simulink model "Assignment_2"  (R2022b)
settings: Solver=FixedStepAuto  StartTime=0.0  StopTime=10.0  FixedStep=1e-3  RelTol=1e-3  EnableMultiTasking=on
undefined symbols (not defined in the file): D0, D1, D10, D11, D12, D13, D2, D3, D5, D6, D8, D9, PTA0, PTA1, PTA2, PTB9, PTC16, PTC17, PTC2, PTC4, PTD0, PTD1, PTD2, PTD3
libraries: frdmk64flib x12
settings Model: ExtModeTrigDuration=5  Creator=aldenluscher  LastModifiedBy=andre
settings OptimizationCC: EnhancedBackFolding=on  PassReuseOutputArgsAs=Individual arguments  ZeroExternalMemoryAtStartup=off  ZeroInternalMemoryAtStartup=off  MaxStackSize=64  OptimizeBlockOrder=speed  DifferentSizesBufferReuse=on  OptimizationCustomize=off  EfficientTunableParamExpr=on
settings DebuggingCC: ParameterTunabilityLossMsg=error
settings HardwareCC: ProdBitPerPointer=32  ProdBitPerSizeT=32  ProdBitPerPtrDiffT=32  ProdLargestAtomicInteger=Long  ProdLargestAtomicFloat=Double  ProdWordSize=32  ProdHWDeviceType=ARM Compatible->ARM Cortex
settings SFSimCC: MATLABDynamicMemAlloc=off
settings RTWCC: Description=Embedded Coder  SystemTargetFile=ert.tlc  HardwareBoard=NXP FRDM-K64F  TLCOptions="-aInlineSetEventsForThisBaseRateFcn=TLC_FALSE -aSuppressMultiTaskScheduler=TLC_FALSE  -aRateBasedStepFcn=0"  TemplateMakefile=ert_default_tmf  Toolchain=GNU Tools for ARM Embedded Processors
settings CodeAppCC: ForceParamTrailComments=on  IgnoreCustomStorageClasses=off  OperatorAnnotations=on  SimulinkDataObjDesc=on  SFDataObjDesc=on  InsertBlockDesc=on
settings ERTTargetCC: ExtModeTransport=4  ExtModeMexFile=sendToCommService

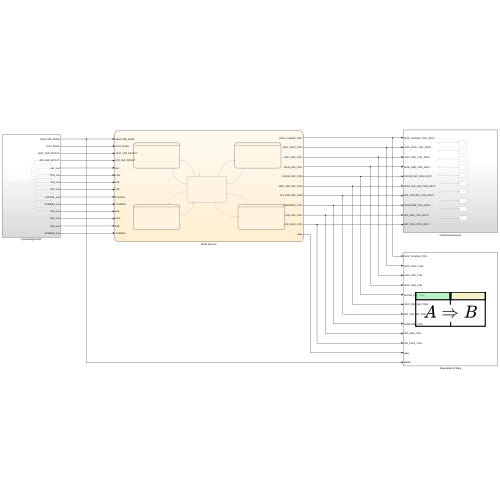
[thumbnail: Simulink's stored preview of the top-level diagram]
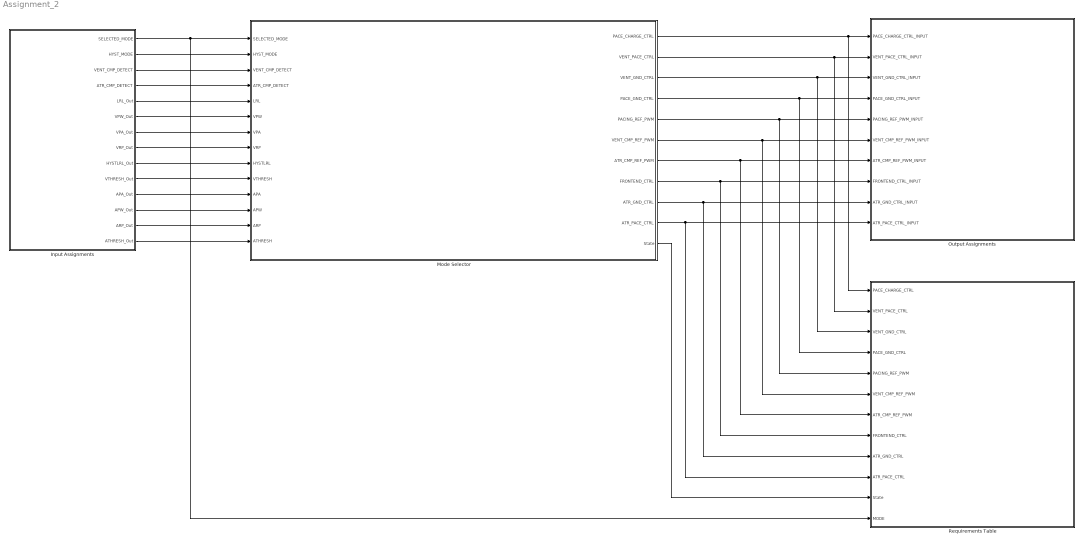
== system Assignment_2 ==
  Input Assignments : Subsystem
  Mode Selector : Stateflow chart  TreatAsAtomicUnit=on
      settings: PortSchema="{\"entries\":[{\"content\":{\"sides\":[{\"content\":{\"connectorIds\":[\"In7\",\"In9\",\"In6\",\"In14\",\"In8\",\"In3\",\"In4\",\"In2\",\"In5\",\"In1\",\"In10\",\"In11\",\"In12\",\"In13\"]},\"type\":\"ConnectorPlacement.EquallySpacedRectSide\",\"uuid\":\"804be3be-5f9e-4b62-b5c8-dc084235daae\"},{\"content\":{\"connectorIds\":[\"Out1\",\"Out2\",\"Out3\",\"Out4\",\"Out5\",\"Out6\",\"Out11\",\"Out7\",\"Out8\",\"Out9\",\"Out10\"],\"side\":\"RIGHT\"},\"type\":\"ConnectorPlacement.EquallySpacedRectSide\",\"uuid\":\"906acfdb-1dc8-44fd-8d51-f28f98719a27\"},{\"content\":{\"connectorIds\":[],\"side\":\"TOP\"},\"type\":\"ConnectorPlacement.EquallySpacedRectSide\",\"uuid\":\"8d057b55-2cbd-487f-8484-177f9fa59c90\"}]},\"type\":\"ConnectorPlacement.EquallySpacedConnector\",\"uuid\":\"d5bd6f86-9a36-412f-a1f0-e96663509123\"}],\"packageUris\":[\"http://schema.mathworks.com/mf0/Connector/R2020b\"],\"version\":\"1.0\"}"
  Output Assignments : Subsystem
  Requirements Table : Requirements Table  TreatAsAtomicUnit=on
  wires:
  Mode Selector/4(PACE_GND_CTRL) -> Requirements Table/4(PACE_GND_CTRL), Output Assignments/4(PACE_GND_CTRL_INPUT)
  Mode Selector/7(FRONTEND_CTRL) -> Output Assignments/8(FRONTEND_CTRL_INPUT), Requirements Table/8(FRONTEND_CTRL)
  Mode Selector/5(PACING_REF_PWM) -> Requirements Table/5(PACING_REF_PWM), Output Assignments/5(PACING_REF_PWM_INPUT)
  Mode Selector/1(PACE_CHARGE_CTRL) -> Requirements Table/1(PACE_CHARGE_CTRL), Output Assignments/1(PACE_CHARGE_CTRL_INPUT)
  Mode Selector/3(VENT_GND_CTRL) -> Requirements Table/3(VENT_GND_CTRL), Output Assignments/3(VENT_GND_CTRL_INPUT)
  Mode Selector/6(VENT_CMP_REF_PWM) -> Requirements Table/6(VENT_CMP_REF_PWM), Output Assignments/6(VENT_CMP_REF_PWM_INPUT)
  Mode Selector/2(VENT_PACE_CTRL) -> Requirements Table/2(VENT_PACE_CTRL), Output Assignments/2(VENT_PACE_CTRL_INPUT)
  Mode Selector/8(ATR_GND_CTRL) -> Output Assignments/9(ATR_GND_CTRL_INPUT), Requirements Table/9(ATR_GND_CTRL)
  Mode Selector/9(ATR_PACE_CTRL) -> Output Assignments/10(ATR_PACE_CTRL_INPUT), Requirements Table/10(ATR_PACE_CTRL)
  Mode Selector/10(State) -> Requirements Table/11(State)
  Mode Selector/11(ATR_CMP_REF_PWM) -> Requirements Table/7(ATR_CMP_REF_PWM), Output Assignments/7(ATR_CMP_REF_PWM_INPUT)
  Input Assignments/1(SELECTED_MODE) -> Requirements Table/12(MODE), Mode Selector/7(SELECTED_MODE)
  Input Assignments/2(HYST_MODE) -> Mode Selector/9(HYST_MODE)
  Input Assignments/3(VENT_CMP_DETECT) -> Mode Selector/6(VENT_CMP_DETECT)
  Input Assignments/4(ATR_CMP_DETECT) -> Mode Selector/14(ATR_CMP_DETECT)
  Input Assignments/5(LRL_Out) -> Mode Selector/8(LRL)
  Input Assignments/6(VPW_Out) -> Mode Selector/3(VPW)
  Input Assignments/7(VPA_Out) -> Mode Selector/4(VPA)
  Input Assignments/8(VRP_Out) -> Mode Selector/2(VRP)
  Input Assignments/9(HYSTLRL_Out) -> Mode Selector/5(HYSTLRL)
  Input Assignments/10(VTHRESH_Out) -> Mode Selector/1(VTHRESH)
  Input Assignments/11(APA_Out) -> Mode Selector/10(APA)
  Input Assignments/12(APW_Out) -> Mode Selector/11(APW)
  Input Assignments/13(ARP_Out) -> Mode Selector/12(ARP)
  Input Assignments/14(ATHRESH_Out) -> Mode Selector/13(ATHRESH)

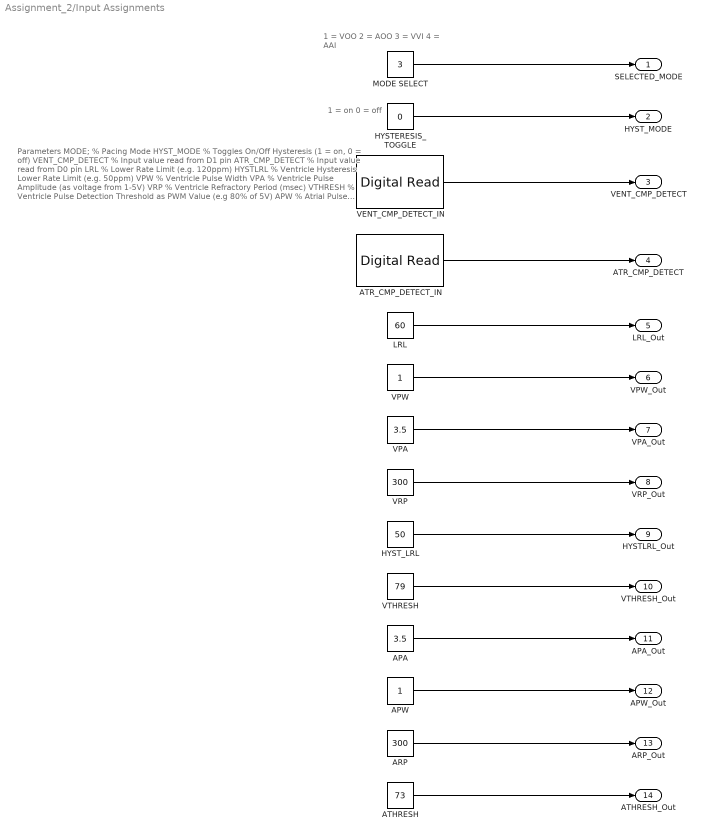
== system Assignment_2/Input Assignments ==
  note: Parameters
      | MODE; 					% Pacing Mode
      | HYST_MODE 			% Toggles On/Off Hysteresis (1 = on, 0 = off)
      | VENT_CMP_DETECT 	% Input value read from D1 pin
      | ATR_CMP_DETECT 		% Input value read from D0 pin
      | LRL 		%  Lower Rate Limit (e.g. 120ppm)
      | HYSTLRL	% Ventricle Hysteresis Lower Rate Limit (e.g. 50ppm)
      | VPW		% Ventricle Pulse Width
      | VPA 		% Ventricle Pulse Amplitude (as voltage from 1-5V)
      | VRP		% Ventricle Refractory Period (msec)
      | VTHRESH 	% Ventricle Pulse Detection Threshold as PWM Value (e.g 80% of 5V)
      | APW		% Atrial Pulse Width
      | APA 		% Atrial Pulse Amplitude (as voltage from 1-5V)
      | ARP 		% Atrial Refractory Period (msec)
      | ATHRESH 	% Atrial Pulse Detection Threshold as a PWM Value (e.g. 80% of 5V)
  note: 1 = VOO
      | 2 = AOO
      | 3 = VVI
      | 4 = AAI
  note: 1 = on
      | 0 = off
  APA : Constant  Value=3.5
  APW : Constant
  ARP : Constant  Value=300
  ATHRESH : Constant  Value=73
  ATR_CMP_DETECT_IN : frdmk64flib/Digital Read  Whichpin=PTC16 (D0)  SampleTime=-1
  HYSTERESIS_TOGGLE : Constant  Value=0
  HYST_LRL : Constant  Value=50
  LRL : Constant  Value=60
  MODE SELECT : Constant  Value=3  OutDataTypeStr=int8
  VENT_CMP_DETECT_IN : frdmk64flib/Digital Read  Whichpin=PTC17 (D1)  SampleTime=-1
  VPA : Constant  Value=3.5
  VPW : Constant
  VRP : Constant  Value=300
  VTHRESH : Constant  Value=79
  SELECTED_MODE : Outport
  HYST_MODE : Outport  Port=2
  VENT_CMP_DETECT : Outport  Port=3
  ATR_CMP_DETECT : Outport  Port=4
  LRL_Out : Outport  Port=5
  VPW_Out : Outport  Port=6
  VPA_Out : Outport  Port=7
  VRP_Out : Outport  Port=8
  HYSTLRL_Out : Outport  Port=9
  VTHRESH_Out : Outport  Port=10
  APA_Out : Outport  Port=11
  APW_Out : Outport  Port=12
  ARP_Out : Outport  Port=13
  ATHRESH_Out : Outport  Port=14
  wires:
  MODE SELECT/1 -> SELECTED_MODE/1
  HYSTERESIS_TOGGLE/1 -> HYST_MODE/1
  VENT_CMP_DETECT_IN/1 -> VENT_CMP_DETECT/1
  ATR_CMP_DETECT_IN/1 -> ATR_CMP_DETECT/1
  LRL/1 -> LRL_Out/1
  VPW/1 -> VPW_Out/1
  VPA/1 -> VPA_Out/1
  VRP/1 -> VRP_Out/1
  HYST_LRL/1 -> HYSTLRL_Out/1
  VTHRESH/1 -> VTHRESH_Out/1
  APA/1 -> APA_Out/1
  APW/1 -> APW_Out/1
  ARP/1 -> ARP_Out/1
  ATHRESH/1 -> ATHRESH_Out/1

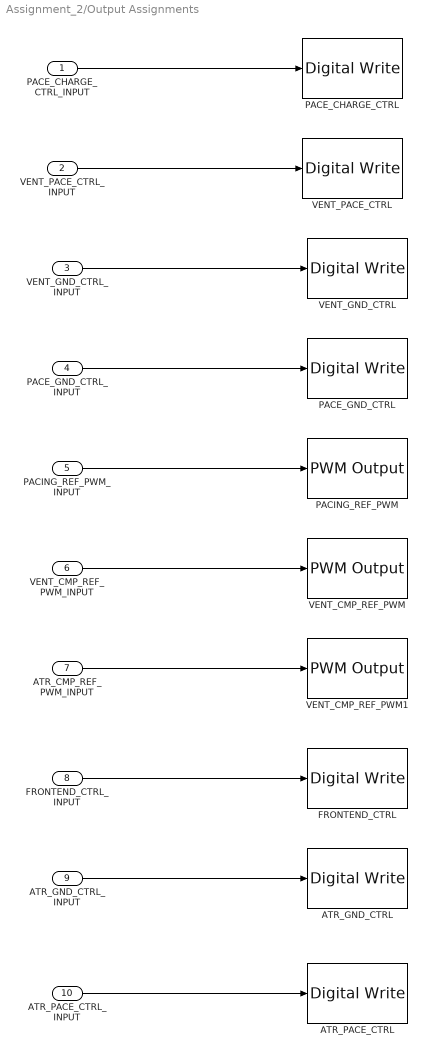
== system Assignment_2/Output Assignments ==
  PACE_CHARGE_CTRL_INPUT : Inport
  VENT_PACE_CTRL_INPUT : Inport  Port=2
  VENT_GND_CTRL_INPUT : Inport  Port=3
  PACE_GND_CTRL_INPUT : Inport  Port=4
  PACING_REF_PWM_INPUT : Inport  Port=5
  VENT_CMP_REF_PWM_INPUT : Inport  Port=6
  ATR_CMP_REF_PWM_INPUT : Inport  Port=7
  FRONTEND_CTRL_INPUT : Inport  Port=8
  ATR_GND_CTRL_INPUT : Inport  Port=9
  ATR_PACE_CTRL_INPUT : Inport  Port=10
  ATR_GND_CTRL : frdmk64flib/Digital Write  Whichpin=PTD2 (D11)
  ATR_PACE_CTRL : frdmk64flib/Digital Write  Whichpin=PTA0 (D8)
  FRONTEND_CTRL : frdmk64flib/Digital Write  Whichpin=PTD1 (D13)
  PACE_CHARGE_CTRL : frdmk64flib/Digital Write  Whichpin=PTB9 (D2)
  PACE_GND_CTRL : frdmk64flib/Digital Write  Whichpin=PTD0 (D10)
  PACING_REF_PWM : frdmk64flib/PWM Output  Whichpin=PTA2 (D5)  InitialFrequency=2000  InitialDutyCycle=0
  VENT_CMP_REF_PWM : frdmk64flib/PWM Output  Whichpin=PTA1 (D3)  InitialFrequency=2000  InitialDutyCycle=0
  VENT_CMP_REF_PWM1 : frdmk64flib/PWM Output  Whichpin=PTC2 (D6)  InitialFrequency=2000  InitialDutyCycle=0
  VENT_GND_CTRL : frdmk64flib/Digital Write  Whichpin=PTD3 (D12)
  VENT_PACE_CTRL : frdmk64flib/Digital Write  Whichpin=PTC4 (D9)
  wires:
  VENT_PACE_CTRL_INPUT/1 -> VENT_PACE_CTRL/1
  PACE_GND_CTRL_INPUT/1 -> PACE_GND_CTRL/1
  PACE_CHARGE_CTRL_INPUT/1 -> PACE_CHARGE_CTRL/1
  PACING_REF_PWM_INPUT/1 -> PACING_REF_PWM/1
  VENT_GND_CTRL_INPUT/1 -> VENT_GND_CTRL/1
  VENT_CMP_REF_PWM_INPUT/1 -> VENT_CMP_REF_PWM/1
  FRONTEND_CTRL_INPUT/1 -> FRONTEND_CTRL/1
  ATR_GND_CTRL_INPUT/1 -> ATR_GND_CTRL/1
  ATR_PACE_CTRL_INPUT/1 -> ATR_PACE_CTRL/1
  ATR_CMP_REF_PWM_INPUT/1 -> VENT_CMP_REF_PWM1/1

== stateflow chart Assignment_2/Requirements Table ==
  (default) -> (junction 1073753187)
  (junction 1073753187) -> (junction 1073753188) : {
      | % SF_REQ_REV_07
      | }
  (junction 1073753188) -> (junction 1073753190) : {
      | % HEADER_ASSIGNMENTS
      |
      | }
  (junction 1073753190) -> (junction 1073753192) : {
      | % START_A_4
      | }
  (junction 1073753192) -> (junction 1073753194) : {
      | }
  (junction 1073753194) -> (junction 1073753196)
  (junction 1073753196) -> (junction 1073753198) : {
      | }
  (junction 1073753198) -> (junction 1073753200) : {
      | % END_A_4
      | }
  (junction 1073753200) -> (junction 1073753202) : {
      | % START_R_40
      | }
  (junction 1073753202) -> (junction 1073753204) : {
      | }
  (junction 1073753204) -> (junction 1073753206)
  (junction 1073753206) -> (junction 1073753208) [order 1] : [(((MODE) == (1)))]
  (junction 1073753206) -> (junction 1073753250) [order 2]
  (junction 1073753208) -> (junction 1073753210) : {
      | reqtable_postcondition((((ATR_PACE_CTRL) == (0))) && (((ATR_GND_CTRL) == (0))) && (((PACING_REF_PWM) >= (0) && (PACING_REF_PWM) <= (100))) && (((VENT_CMP_REF_PWM) >= (0) && (VENT_CMP_REF_PWM) <= (100))) && (((ATR_CMP_REF_PWM) >= (0) && (ATR_CMP_REF_PWM) <= (100))) && (((FRONTEND_CTRL) == (0))), 'R:1');
      |
      |
      | }
  (junction 1073753210) -> (junction 1073753212) : {
      | }
  (junction 1073753212) -> (junction 1073753214) : {
      | % START_R_16
      | }
  (junction 1073753214) -> (junction 1073753216) : {
      | }
  (junction 1073753216) -> (junction 1073753218)
  (junction 1073753218) -> (junction 1073753220) [order 1] : [(((State) == (0)))]
  (junction 1073753218) -> (junction 1073753226) [order 2]
  (junction 1073753220) -> (junction 1073753222) : {
      | reqtable_postcondition((((PACE_CHARGE_CTRL) == (1))) && (((PACE_GND_CTRL) == (1))) && (((VENT_PACE_CTRL) == (0))) && (((VENT_GND_CTRL) == (1))), 'R:1.1');
      |
      |
      | }
  (junction 1073753222) -> (junction 1073753224) : {
      | }
  (junction 1073753224) -> (junction 1073753226)
  (junction 1073753226) -> (junction 1073753228)
  (junction 1073753228) -> (junction 1073753230) : {
      | % END_R_16
      | }
  (junction 1073753230) -> (junction 1073753232) : {
      | % START_R_22
      | }
  (junction 1073753232) -> (junction 1073753234) : {
      | }
  (junction 1073753234) -> (junction 1073753236)
  (junction 1073753236) -> (junction 1073753238) [order 1] : [(((State) == (1)))]
  (junction 1073753236) -> (junction 1073753244) [order 2]
  (junction 1073753238) -> (junction 1073753240) : {
      | reqtable_postcondition((((PACE_CHARGE_CTRL) == (0))) && (((PACE_GND_CTRL) == (1))) && (((VENT_PACE_CTRL) == (1))) && (((VENT_GND_CTRL) == (0))), 'R:1.2');
      |
      |
      | }
  (junction 1073753240) -> (junction 1073753242) : {
      | }
  (junction 1073753242) -> (junction 1073753244)
  (junction 1073753244) -> (junction 1073753246)
  (junction 1073753246) -> (junction 1073753248) : {
      | % END_R_22
      | }
  (junction 1073753248) -> (junction 1073753250)
  (junction 1073753250) -> (junction 1073753252)
  (junction 1073753252) -> (junction 1073753254) : {
      | % END_R_40
      | }
  (junction 1073753254) -> (junction 1073753256) : {
      | % START_R_43
      | }
  (junction 1073753256) -> (junction 1073753258) : {
      | }
  (junction 1073753258) -> (junction 1073753260)
  (junction 1073753260) -> (junction 1073753262) [order 1] : [(((MODE) == (2)))]
  (junction 1073753260) -> (junction 1073753304) [order 2]
  (junction 1073753262) -> (junction 1073753264) : {
      | reqtable_postcondition((((VENT_PACE_CTRL) == (0))) && (((VENT_GND_CTRL) == (0))) && (((PACING_REF_PWM) >= (0) && (PACING_REF_PWM) <= (100))) && (((VENT_CMP_REF_PWM) >= (0) && (VENT_CMP_REF_PWM) <= (100))) && (((ATR_CMP_REF_PWM) >= (0) && (ATR_CMP_REF_PWM) <= (100))) && (((FRONTEND_CTRL) == (0))), 'R:2');
      |
      |
      | }
  (junction 1073753264) -> (junction 1073753266) : {
      | }
  (junction 1073753266) -> (junction 1073753268) : {
      | % START_R_25
      | }
  (junction 1073753268) -> (junction 1073753270) : {
      | }
  (junction 1073753270) -> (junction 1073753272)
  (junction 1073753272) -> (junction 1073753274) [order 1] : [(((State) == (0)))]
  (junction 1073753272) -> (junction 1073753280) [order 2]
  (junction 1073753274) -> (junction 1073753276) : {
      | reqtable_postcondition((((PACE_CHARGE_CTRL) == (1))) && (((PACE_GND_CTRL) == (1))) && (((ATR_PACE_CTRL) == (0))) && (((ATR_GND_CTRL) == (1))), 'R:2.1');
      |
      |
      | }
  (junction 1073753276) -> (junction 1073753278) : {
      | }
  (junction 1073753278) -> (junction 1073753280)
  (junction 1073753280) -> (junction 1073753282)
  (junction 1073753282) -> (junction 1073753284) : {
      | % END_R_25
      | }
  (junction 1073753284) -> (junction 1073753286) : {
      | % START_R_28
      | }
  (junction 1073753286) -> (junction 1073753288) : {
      | }
  (junction 1073753288) -> (junction 1073753290)
  (junction 1073753290) -> (junction 1073753292) [order 1] : [(((State) == (1)))]
  (junction 1073753290) -> (junction 1073753298) [order 2]
  (junction 1073753292) -> (junction 1073753294) : {
      | reqtable_postcondition((((PACE_CHARGE_CTRL) == (0))) && (((PACE_GND_CTRL) == (1))) && (((ATR_PACE_CTRL) == (1))) && (((ATR_GND_CTRL) == (0))), 'R:2.2');
      |
      |
      | }
  (junction 1073753294) -> (junction 1073753296) : {
      | }
  (junction 1073753296) -> (junction 1073753298)
  (junction 1073753298) -> (junction 1073753300)
  (junction 1073753300) -> (junction 1073753302) : {
      | % END_R_28
      | }
  (junction 1073753302) -> (junction 1073753304)
  (junction 1073753304) -> (junction 1073753306)
  (junction 1073753306) -> (junction 1073753308) : {
      | % END_R_43
      | }
  (junction 1073753308) -> (junction 1073753310) : {
      | % START_R_61
      | }
  (junction 1073753310) -> (junction 1073753312) : {
      | }
  (junction 1073753312) -> (junction 1073753314)
  (junction 1073753314) -> (junction 1073753316) [order 1] : [(((MODE) == (3)))]
  (junction 1073753314) -> (junction 1073753376) [order 2]
  (junction 1073753316) -> (junction 1073753318) : {
      | reqtable_postcondition((((ATR_PACE_CTRL) == (0))) && (((ATR_GND_CTRL) == (0))) && (((PACING_REF_PWM) >= (0) && (PACING_REF_PWM) <= (100))) && (((VENT_CMP_REF_PWM) >= (0) && (VENT_CMP_REF_PWM) <= (100))) && (((ATR_CMP_REF_PWM) >= (0) && (ATR_CMP_REF_PWM) <= (100))) && (((FRONTEND_CTRL) == (1))), 'R:3');
      |
      |
      | }
  (junction 1073753318) -> (junction 1073753320) : {
      | }
  (junction 1073753320) -> (junction 1073753322) : {
      | % START_R_64
      | }
  (junction 1073753322) -> (junction 1073753324) : {
      | }
  (junction 1073753324) -> (junction 1073753326)
  (junction 1073753326) -> (junction 1073753328) [order 1] : [(((State) == (0)))]
  (junction 1073753326) -> (junction 1073753334) [order 2]
  (junction 1073753328) -> (junction 1073753330) : {
      | reqtable_postcondition((((PACE_CHARGE_CTRL) == (1))) && (((PACE_GND_CTRL) == (1))) && (((VENT_PACE_CTRL) == (0))) && (((VENT_GND_CTRL) == (1))), 'R:3.1');
      |
      |
      | }
  (junction 1073753330) -> (junction 1073753332) : {
      | }
  (junction 1073753332) -> (junction 1073753334)
  (junction 1073753334) -> (junction 1073753336)
  (junction 1073753336) -> (junction 1073753338) : {
      | % END_R_64
      | }
  (junction 1073753338) -> (junction 1073753340) : {
      | % START_R_67
      | }
  (junction 1073753340) -> (junction 1073753342) : {
      | }
  (junction 1073753342) -> (junction 1073753344)
  (junction 1073753344) -> (junction 1073753346) [order 1] : [(((State) == (1)))]
  (junction 1073753344) -> (junction 1073753352) [order 2]
  (junction 1073753346) -> (junction 1073753348) : {
      | reqtable_postcondition((((PACE_CHARGE_CTRL) == (0))) && (((PACE_GND_CTRL) == (1))) && (((VENT_PACE_CTRL) == (1))) && (((VENT_GND_CTRL) == (0))), 'R:3.2');
      |
      |
      | }
  (junction 1073753348) -> (junction 1073753350) : {
      | }
  (junction 1073753350) -> (junction 1073753352)
  (junction 1073753352) -> (junction 1073753354)
  (junction 1073753354) -> (junction 1073753356) : {
      | % END_R_67
      | }
  (junction 1073753356) -> (junction 1073753358) : {
      | % START_R_73
      | }
  (junction 1073753358) -> (junction 1073753360) : {
      | }
  (junction 1073753360) -> (junction 1073753362)
  (junction 1073753362) -> (junction 1073753364) [order 1] : [(((State) == (2)))]
  (junction 1073753362) -> (junction 1073753370) [order 2]
  (junction 1073753364) -> (junction 1073753366) : {
      | reqtable_postcondition((((PACE_CHARGE_CTRL) == (1))) && (((PACE_GND_CTRL) == (1))) && (((VENT_PACE_CTRL) == (0))) && (((VENT_GND_CTRL) == (1))), 'R:3.3');
      |
      |
      | }
  (junction 1073753366) -> (junction 1073753368) : {
      | }
  (junction 1073753368) -> (junction 1073753370)
  (junction 1073753370) -> (junction 1073753372)
  (junction 1073753372) -> (junction 1073753374) : {
      | % END_R_73
      | }
  (junction 1073753374) -> (junction 1073753376)
  (junction 1073753376) -> (junction 1073753378)
  (junction 1073753378) -> (junction 1073753380) : {
      | % END_R_61
      | }
  (junction 1073753380) -> (junction 1073753382) : {
      | % START_R_52
      | }
  (junction 1073753382) -> (junction 1073753384) : {
      | }
  (junction 1073753384) -> (junction 1073753386)
  (junction 1073753386) -> (junction 1073753388) [order 1] : [(((MODE) == (4)))]
  (junction 1073753386) -> (junction 1073753448) [order 2]
  (junction 1073753388) -> (junction 1073753390) : {
      | reqtable_postcondition((((VENT_PACE_CTRL) == (0))) && (((VENT_GND_CTRL) == (0))) && (((PACING_REF_PWM) >= (0) && (PACING_REF_PWM) <= (100))) && (((VENT_CMP_REF_PWM) >= (0) && (VENT_CMP_REF_PWM) <= (100))) && (((ATR_CMP_REF_PWM) >= (0) && (ATR_CMP_REF_PWM) <= (100))) && (((FRONTEND_CTRL) == (1))), 'R:4');
      |
      |
      | }
  (junction 1073753390) -> (junction 1073753392) : {
      | }
  (junction 1073753392) -> (junction 1073753394) : {
      | % START_R_55
      | }
  (junction 1073753394) -> (junction 1073753396) : {
      | }
  (junction 1073753396) -> (junction 1073753398)
  (junction 1073753398) -> (junction 1073753400) [order 1] : [(((State) == (0)))]
  (junction 1073753398) -> (junction 1073753406) [order 2]
  (junction 1073753400) -> (junction 1073753402) : {
      | reqtable_postcondition((((PACE_CHARGE_CTRL) == (1))) && (((PACE_GND_CTRL) == (1))) && (((ATR_PACE_CTRL) == (0))) && (((ATR_GND_CTRL) == (1))), 'R:4.1');
      |
      |
      | }
  (junction 1073753402) -> (junction 1073753404) : {
      | }
  (junction 1073753404) -> (junction 1073753406)
  (junction 1073753406) -> (junction 1073753408)
  (junction 1073753408) -> (junction 1073753410) : {
      | % END_R_55
      | }
  (junction 1073753410) -> (junction 1073753412) : {
      | % START_R_58
      | }
  (junction 1073753412) -> (junction 1073753414) : {
      | }
  (junction 1073753414) -> (junction 1073753416)
  (junction 1073753416) -> (junction 1073753418) [order 1] : [(((State) == (1)))]
  (junction 1073753416) -> (junction 1073753424) [order 2]
  (junction 1073753418) -> (junction 1073753420) : {
      | reqtable_postcondition((((PACE_CHARGE_CTRL) == (0))) && (((PACE_GND_CTRL) == (1))) && (((ATR_PACE_CTRL) == (1))) && (((ATR_GND_CTRL) == (0))), 'R:4.2');
      |
      |
      | }
  (junction 1073753420) -> (junction 1073753422) : {
      | }
  (junction 1073753422) -> (junction 1073753424)
  (junction 1073753424) -> (junction 1073753426)
  (junction 1073753426) -> (junction 1073753428) : {
      | % END_R_58
      | }
  (junction 1073753428) -> (junction 1073753430) : {
      | % START_R_70
      | }
  (junction 1073753430) -> (junction 1073753432) : {
      | }
  (junction 1073753432) -> (junction 1073753434)
  (junction 1073753434) -> (junction 1073753436) [order 1] : [(((State) == (2)))]
  (junction 1073753434) -> (junction 1073753442) [order 2]
  (junction 1073753436) -> (junction 1073753438) : {
      | reqtable_postcondition((((PACE_CHARGE_CTRL) == (1))) && (((PACE_GND_CTRL) == (1))) && (((ATR_PACE_CTRL) == (0))) && (((ATR_GND_CTRL) == (1))), 'R:4.3');
      |
      |
      | }
  (junction 1073753438) -> (junction 1073753440) : {
      | }
  (junction 1073753440) -> (junction 1073753442)
  (junction 1073753442) -> (junction 1073753444)
  (junction 1073753444) -> (junction 1073753446) : {
      | % END_R_70
      | }
  (junction 1073753446) -> (junction 1073753448)
  (junction 1073753448) -> (junction 1073753450)
  (junction 1073753450) -> (junction 1073753452) : {
      | % END_R_52
      | }
  data: PACE_CHARGE_CTRL input; VENT_PACE_CTRL input; VENT_GND_CTRL input; PACE_GND_CTRL input; PACING_REF_PWM input; VENT_CMP_REF_PWM input; ATR_CMP_REF_PWM input; FRONTEND_CTRL input; ATR_GND_CTRL input; ATR_PACE_CTRL input; State input int8 [0..2]; MODE input

== stateflow chart Assignment_2/Mode Selector ==
  state VOO
    state Pacing_
      PACE_CHARGE_CTRL = 0;
      PACE_GND_CTRL = 1;
      VENT_GND_CTRL = 0;
      VENT_PACE_CTRL = 1;
      State = 1;
    state Charging_
      State = 0;
      PACING_REF_PWM = 100*(VPA/5); % Ventricular Pulse Amplitude
      PACING_PERIOD = (60000/LRL); % Pacing Period
      PACE_CHARGE_CTRL = 1;
      PACE_GND_CTRL = 1;
      VENT_GND_CTRL = 1;
      VENT_PACE_CTRL = 0;
      ATR_PACE_CTRL = 0;
      ATR_GND_CTRL = 0;
    (default) -> VOO.Charging_
    VOO.Charging_ -> VOO.Pacing_ : after(PACING_PERIOD-VPW,msec)
        | %Charging time = Pacing Period - Pulse Width
    VOO.Pacing_ -> VOO.Charging_ : after(VPW,msec)
        | %Pacing time = Ventricle Pulse Width
  state VVI
    state Timing_Natural_PW_in_msec_
      NAT_PW=NAT_PW+1;
    state Refractory_Period_
      PACE_CHARGE_CTRL = 1;
      PACE_GND_CTRL = 1;
      VENT_GND_CTRL = 1;
      VENT_PACE_CTRL = 0;
      State = 2;
    state Charging_
      PACING_REF_PWM = 100*(VPA/5); %Pulse Amplitude
      PACING_PERIOD = (60000/LRL); %Normal Pacing Period
      HYST_PERIOD = (60000/HYSTLRL); %Hysteresis Pacing Period
      PACE_CHARGE_CTRL = 1;
      PACE_GND_CTRL = 1;
      VENT_GND_CTRL = 1;
      VENT_PACE_CTRL = 0;
      VENT_CMP_REF_PWM = VTHRESH; % Ventricle Sensing Threshold
      FRONTEND_CTRL = 1; %Sensing On
      NAT_PW = 0; % Natural Pulse Width
      TOTAL_NAT_PW = 0; % Sum of Natural Pulse
      PACE_PW = 0; % Pacemaker Pulse Width
      ARTIFICIAL = 0; % Flag to determine if a pulse was natural or artificial,
      % only has an effect when hysteresis is enabled
      State = 0;
    state Pacing_
      PACE_CHARGE_CTRL = 0;
      PACE_GND_CTRL = 1;
      VENT_GND_CTRL = 0;
      VENT_PACE_CTRL = 1;
      State = 1;
    state Setting_Initial_Period_
      PERIOD = (60000/LRL);
      % Period for each
      % pulse, initally set to the
      % normal PACING_PERIOD
      % but can be re-assigned to
      % the HYST_PERIOD if
      % hysteresis is enabled and
      % triggered
      ATR_PACE_CTRL = 0;
      ATR_GND_CTRL = 0;
      % Set ATR_PACE and
      % GND_CTRL to disabled
      % incase they were left enabled
      % from the last state
    VVI.Timing_Natural_PW_in_msec_ -> VVI.Timing_Natural_PW_in_msec_ [order 2] : after(1,msec)
        | % time the natural pulse in msec
    VVI.Refractory_Period_ -> VVI.Timing_Natural_PW_in_msec_ [order 1] : [VENT_CMP_DETECT==1]{ARTIFICIAL = 0}
        | % if a natural pulse arrives while
        | % in the refractory period, the last pulse was not
        | % from the pulsemaker, and start timing the natural pulse
    VVI.Timing_Natural_PW_in_msec_ -> VVI.Refractory_Period_ [order 1] : [VENT_CMP_DETECT==0]{TOTAL_NAT_PW = TOTAL_NAT_PW + NAT_PW}
        | % when the natural pulse ends add the pulsewidth of the natural pulse to the
        | % total pulsewidth of all natural pulses that have arrived while since we last
        | % paced the pacemaker
    VVI.Refractory_Period_ -> (junction 80) [order 2] : [after(VRP-PACE_PW-TOTAL_NAT_PW,msec) || VRP-PACE_PW-TOTAL_NAT_PW <= 0]
        | % after VRP-PACE_PW-TOTAL_NAT_PW then charge
        | % OR if VRP-PACE_PW-TOTAL_NAT_PW has fallen
        | % beneath the VRP duration
    (junction 80) -> VVI.Charging_ [order 1] : [HYST_MODE == 1 && ARTIFICIAL == 0]{PERIOD = HYST_PERIOD}
        | % if hysteresis mode is on and the last pulse was a natural
        | % pulse then the pacing period for the next pulse is the HYST_PERIOD
    (junction 80) -> VVI.Charging_ [order 3] : [HYST_MODE==0]
        | % if hysteresis mode is off
    (junction 80) -> VVI.Charging_ [order 2] : [HYST_MODE == 1 && ARTIFICIAL == 1]{PERIOD = PACING_PERIOD}
        | % if hysteresis mode is on and the last pulse was sent
        | % by the pacemaker then the next pulse is the normal PACING_PERIOD
    (junction 77) -> VVI.Refractory_Period_ [order 2] : [VENT_CMP_DETECT == 1]
        | % if an incoming pulse is detected
    VVI.Pacing_ -> VVI.Refractory_Period_ : after(VPW,msec){PACE_PW = VPW, ARTIFICIAL = 1}
        | % pace for duration of VPW
    (default) -> VVI.Setting_Initial_Period_
    VVI.Charging_ -> (junction 77)
    (junction 77) -> VVI.Pacing_ [order 1] : after(PERIOD-VPW-VRP,msec)[VENT_CMP_DETECT == 0]
        | % after PERIOD-VPW-VRP if no pulse is detected then pace
    VVI.Setting_Initial_Period_ -> VVI.Charging_
  state PACING_MODE_ENTRY_POINT_
    % Selects which mode to enter into
  state AOO
    state Pacing_
      PACE_CHARGE_CTRL = 0;
      PACE_GND_CTRL = 1;
      ATR_GND_CTRL = 0;
      ATR_PACE_CTRL = 1;
      State = 1;
    state Charging_
      PACING_REF_PWM = 100*(APA/5); % Atrial Pulse Amplitude
      PACING_PERIOD = (60000/LRL); % Pacing Period
      PACE_CHARGE_CTRL = 1;
      PACE_GND_CTRL = 1;
      ATR_GND_CTRL = 1;
      ATR_PACE_CTRL = 0;
      VENT_GND_CTRL = 0;
      VENT_PACE_CTRL = 0;
      State = 0;
    (default) -> AOO.Charging_
    AOO.Charging_ -> AOO.Pacing_ : after(PACING_PERIOD-APW,msec)
        | %Charging time = Pacing Period - Pulse Width
    AOO.Pacing_ -> AOO.Charging_ : after(APW,msec)
        | %Pacing time = Atrial Pulse Width
  state AAI
    state Timing_Natural_PW_in_msec_
      NAT_PW=NAT_PW+1;
    state Refractory_Period_
      PACE_CHARGE_CTRL = 1;
      PACE_GND_CTRL = 1;
      ATR_GND_CTRL = 1;
      ATR_PACE_CTRL = 0;
      State = 2;
    state Charging_
      PACING_REF_PWM = 100*(APA/5); %Pulse Amplitude
      PACING_PERIOD = (60000/LRL); %Normal Pacing Period
      HYST_PERIOD = (60000/HYSTLRL); %Hysteresis Pacing Period
      PACE_CHARGE_CTRL = 1;
      PACE_GND_CTRL = 1;
      ATR_GND_CTRL = 1;
      ATR_PACE_CTRL = 0;
      ATR_CMP_REF_PWM = ATHRESH; % Atrial Sensing Threshold
      FRONTEND_CTRL = 1; %Sensing On
      NAT_PW = 0; % Natural Pulse Width
      TOTAL_NAT_PW = 0; % Sum of Natural Pulse
      PACE_PW = 0; % Pacemaker Pulse Width
      ARTIFICIAL = 0; % Flag to determine if a pulse was natural or artificial,
      % only has an effect when hysteresis is enabled
      State = 0;
    state Pacing_
      PACE_CHARGE_CTRL = 0;
      PACE_GND_CTRL = 1;
      ATR_GND_CTRL = 0;
      ATR_PACE_CTRL = 1;
      State = 1;
    state Setting_Initial_Period_
      PERIOD = (60000/LRL);
      % Period for each
      % pulse, initally set to the
      % normal PACING_PERIOD
      % but can be re-assigned to
      % the HYST_PERIOD if
      % hysteresis is enabled and
      % triggered
      VENT_PACE_CTRL = 0;
      VENT_GND_CTRL = 0;
      % Set VENT_PACE and
      % GND_CTRL to disabled
      % incase they were left enabled
      % from the last state
    AAI.Timing_Natural_PW_in_msec_ -> AAI.Timing_Natural_PW_in_msec_ [order 2] : after(1,msec)
        | % time the natural pulse in msec
    AAI.Timing_Natural_PW_in_msec_ -> AAI.Refractory_Period_ [order 1] : [ATR_CMP_DETECT==0]{TOTAL_NAT_PW = TOTAL_NAT_PW + NAT_PW}
        | % when the natural pulse ends add the pulsewidth of the natural pulse to the
        | % total pulsewidth of all natural pulses that have arrived while since we last
        | % paced the pacemaker
    AAI.Refractory_Period_ -> AAI.Timing_Natural_PW_in_msec_ [order 1] : [ATR_CMP_DETECT==1]{ARTIFICIAL = 0}
        | % if a natural pulse arrives while
        | % in the refractory period, the last pulse was not
        | % from the pulsemaker, and start timing the natural pulse
    AAI.Refractory_Period_ -> (junction 172) [order 2] : [after(ARP-PACE_PW-TOTAL_NAT_PW,msec) || ARP-PACE_PW-TOTAL_NAT_PW <= 0]
        | % after ARP-PACE_PW-TOTAL_NAT_PW then charge
        | % OR if ARP-PACE_PW-TOTAL_NAT_PW has fallen
        | % beneath the ARP duration
    (junction 172) -> AAI.Charging_ [order 1] : [HYST_MODE == 1 && ARTIFICIAL == 0]{PERIOD = HYST_PERIOD}
        | % if hysteresis mode is on and the last pulse was a natural
        | % pulse then the pacing period for the next pulse is the HYST_PERIOD
    (junction 172) -> AAI.Charging_ [order 3] : [HYST_MODE==0]
        | % if hysteresis mode is off
    (junction 172) -> AAI.Charging_ [order 2] : [HYST_MODE == 1 && ARTIFICIAL == 1]{PERIOD = PACING_PERIOD}
        | % if hysteresis mode is on and the last pulse was sent
        | % by the pacemaker then the next pulse is the normal PACING_PERIOD
    (junction 173) -> AAI.Refractory_Period_ [order 2] : [ATR_CMP_DETECT == 1]
        | % if an incoming pulse is detected
    AAI.Pacing_ -> AAI.Refractory_Period_ : after(APW,msec){PACE_PW = APW, ARTIFICIAL = 1}
        | % pace for duration of APW
    (default) -> AAI.Setting_Initial_Period_
    AAI.Charging_ -> (junction 173)
    (junction 173) -> AAI.Pacing_ [order 1] : after(PERIOD-APW-ARP,msec)[ATR_CMP_DETECT == 0]
        | % after PERIOD-APW-ARP if no pulse is detected then pace
    AAI.Setting_Initial_Period_ -> AAI.Charging_
  PACING_MODE_ENTRY_POINT_ -> VOO [order 2] : [SELECTED_MODE==1]
  PACING_MODE_ENTRY_POINT_ -> VVI [order 1] : [SELECTED_MODE==3]
  VOO -> PACING_MODE_ENTRY_POINT_ : [SELECTED_MODE~=1]
  VVI -> PACING_MODE_ENTRY_POINT_ : [SELECTED_MODE~=3]
  (default) -> PACING_MODE_ENTRY_POINT_
  PACING_MODE_ENTRY_POINT_ -> AOO [order 3] : [SELECTED_MODE==2]
  AAI -> PACING_MODE_ENTRY_POINT_ : [SELECTED_MODE~=4]
  AOO -> PACING_MODE_ENTRY_POINT_ : [SELECTED_MODE~=2]
  PACING_MODE_ENTRY_POINT_ -> AAI [order 4] : [SELECTED_MODE==4]
  data: PACE_CHARGE_CTRL output int8; VENT_PACE_CTRL output int8; VENT_GND_CTRL output int8; PACE_GND_CTRL output int8; PACING_REF_PWM output; VENT_CMP_REF_PWM output; PACING_PERIOD local; PERIOD local; HYST_PERIOD local; FRONTEND_CTRL output int8; NAT_PW local; TOTAL_NAT_PW local; PACE_PW local; VTHRESH input; VRP input; VPW input; VPA input; HYSTLRL input; VENT_CMP_DETECT input; SELECTED_MODE input; LRL input; HYST_MODE input; ARTIFICIAL local; ATR_GND_CTRL output int8; ATR_PACE_CTRL output int8; APA input; APW input; State output int8 [0..2]; ARP input; ATHRESH input; ATR_CMP_DETECT input; ATR_CMP_REF_PWM output
